simulink library "Lib_PF_LineAC_TMATS"  (R2017a)
settings: Solver=ode45  StartTime=0.0  StopTime=10.0  RelTol=1e-3  EnableMultiTasking=on
Description:
  | Thomas Modules
settings Model: Creator=jwchapm2  LastModifiedBy=glthoma1
settings DataIOCC: LimitDataPoints=on  SaveFormat=Array
settings OptimizationCC: ExpressionDepthLimit=2147483647  LifeSpan=inf
settings DebuggingCC: UnderspecifiedInitializationDetection=Classic  MergeDetectMultiDrivingBlocksExec=none  SolverPrmCheckMsg=warning  StateNameClashWarn=warning  SFUnexpectedBacktrackingDiag=warning  SFNoUnconditionalDefaultTransitionDiag=warning  SFExecutionAtInitializationDiag=none
settings HardwareCC: ProdBitPerPointer=32  ProdBitPerSizeT=32  ProdBitPerPtrDiffT=32  ProdLargestAtomicFloat=None  ProdIntDivRoundTo=Undefined  ProdEndianess=Unspecified  ProdWordSize=32  ProdHWDeviceType=32-bit Generic
settings ModelReferenceCC: PropagateSignalLabelsOutOfModel=off
settings GRTTargetCC: TargetLangStandard=C89/C90 (ANSI)  GeneratePreprocessorConditionals=Disable all
settings ConfigComp: CovMetricSettings=dw  CovHtmlReporting=on  CovSaveCumulativeToWorkspaceVar=on  CovSaveSingleToWorkspaceVar=on  CovExternalEMLEnable=off

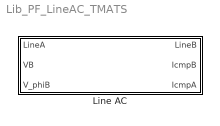
== system Lib_PF_LineAC_TMATS ==
  Line AC : Subsystem  mask{R_M=100, X_M=0.015, Z2R_M=0.015, Z2X_M=0.015}
      mask prompts: R_M "R_M - Z Resistance"; X_M "X_M - Z Reactance"; Z2R_M "Z2R_M - Z_2 Resistance"; Z2X_M "Z2X_M - Z_2 Reactance"
      mask Display:
      | fprintf('Z: R + jX\n %g + j%g\n Z_2: R + jX\n%g + j%g',R_M, X_M,Z2R_M, Z2X_M)
      | port_label('input',1,'VA')
      | port_label('input',2,'VBg')
      | port_label('input',3,'phiBg')
      | port_label('output',1,'VB')
      | port_label('output',2,'IcB')
      | port_label('output',3,'IcA')

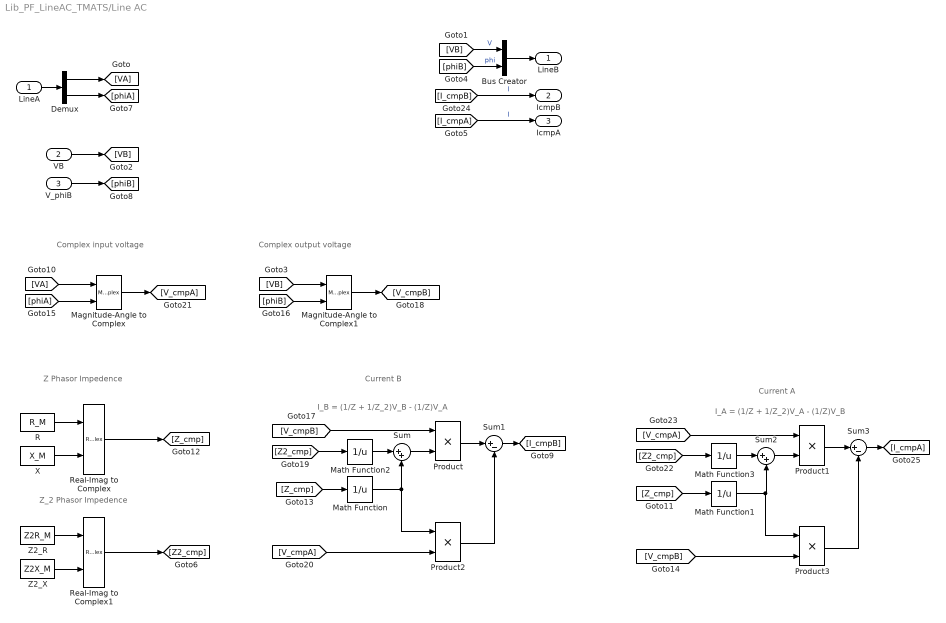
== system Lib_PF_LineAC_TMATS/Line AC ==
  note: I_B = (1/Z + 1/Z_2)V_B - (1/Z)V_A
  note: Complex output voltage
  note: Complex input voltage
  note: Z Phasor Impedence
  note: Current B
  note: Z_2 Phasor Impedence
  note: Current A
  note: I_A = (1/Z + 1/Z_2)V_A - (1/Z)V_B
  LineA : Inport
  VB : Inport  Port=2
  V_phiB : Inport  Port=3
  Bus Creator : BusCreator  Inputs=2
  Demux : Demux  Outputs=2
  Magnitude-Angle to Complex : MagnitudeAngleToComplex
  Magnitude-Angle to Complex1 : MagnitudeAngleToComplex
  Math Function{,1..3} (4 alike) : Math  Operator=reciprocal  SaturateOnIntegerOverflow=on
  Product{,1..3} (4 alike) : Product
  R : Constant  Value=R_M
  Real-Imag to Complex : RealImagToComplex
  Real-Imag to Complex1 : RealImagToComplex
  Sum : Sum  Inputs=|++
  Sum1 : Sum  Inputs=|+-
  Sum2 : Sum  Inputs=|++
  Sum3 : Sum  Inputs=|+-
  X : Constant  Value=X_M
  Z2_R : Constant  Value=Z2R_M
  Z2_X : Constant  Value=Z2X_M
  LineB : Outport
  IcmpB : Outport  Port=2
  IcmpA : Outport  Port=3
  wires:
  Demux/1 -> [VA]
  [phiB] -> Bus Creator/2  "phi"
  [I_cmpA] -> IcmpA/1  "I"
  V_phiB/1 -> [phiB]
  Demux/2 -> [phiA]
  LineA/1 -> Demux/1
  VB/1 -> [VB]
  [VB] -> Bus Creator/1  "V"
  Bus Creator/1 -> LineB/1
  [VA] -> Magnitude-Angle to Complex/1
  [phiA] -> Magnitude-Angle to Complex/2
  Magnitude-Angle to Complex/1 -> [V_cmpA]
  [VB] -> Magnitude-Angle to Complex1/1
  Magnitude-Angle to Complex1/1 -> [V_cmpB]
  [phiB] -> Magnitude-Angle to Complex1/2
  R/1 -> Real-Imag to Complex/1
  X/1 -> Real-Imag to Complex/2
  Real-Imag to Complex/1 -> [Z_cmp]
  [V_cmpB] -> Product/1
  [Z_cmp] -> Math Function/1
  Product/1 -> Sum1/1
  Math Function/1 -> Product2/1, Sum/2
  Z2_R/1 -> Real-Imag to Complex1/1
  Z2_X/1 -> Real-Imag to Complex1/2
  Real-Imag to Complex1/1 -> [Z2_cmp]
  [I_cmpB] -> IcmpB/1  "I"
  Sum/1 -> Product/2
  [Z2_cmp] -> Math Function2/1
  Math Function2/1 -> Sum/1
  Sum1/1 -> [I_cmpB]
  [V_cmpA] -> Product2/2
  Product2/1 -> Sum1/2
  [V_cmpA] -> Product1/1
  [Z_cmp] -> Math Function1/1
  Product1/1 -> Sum3/1
  Math Function1/1 -> Sum2/2, Product3/1
  Sum2/1 -> Product1/2
  [Z2_cmp] -> Math Function3/1
  Math Function3/1 -> Sum2/1
  Sum3/1 -> [I_cmpA]
  [V_cmpB] -> Product3/2
  Product3/1 -> Sum3/2
